simulink model "mpcACCsystem"  (R2023a)
settings: Solver=FixedStepAuto  StartTime=0.0  StopTime=T  RelTol=1e-3
values from neighbouring files (symbols this model uses):
  t_gap = 1.4    [AdaptiveCruiseControlExample.m]
  Ts = 0.1    [AdaptiveCruiseControlExample.m]
  v0_ego = 20    [AdaptiveCruiseControlExample.m]
  v0_lead = 25    [AdaptiveCruiseControlExample.m]
  v_set = 30    [AdaptiveCruiseControlExample.m]
  x0_ego = 10    [AdaptiveCruiseControlExample.m]
  x0_lead = 50    [AdaptiveCruiseControlExample.m]
undefined symbols (not defined in the file or in its folder): MinVelocity
libraries: mpcsigdimcheck_private x10, mpclib x1
settings Model: Creator=The MathWorks, Inc.  LastModifiedBy=15359
settings SolverCC: AlgebraicLoopSolver=TrustRegion
settings DataIOCC: ReturnWorkspaceOutputs=off
settings DebuggingCC: UnconnectedInputMsg=warning  UnconnectedOutputMsg=warning  UnconnectedLineMsg=warning  ArithmeticOperatorsInVariantConditions=warning
settings ModelReferenceCC: EnableRefExpFcnMdlSchedulingChecks=on
settings SFSimCC: SimUseLocalCustomCode=off  CustomCodeUndefinedFunction=UseInterfaceOnly
settings RTWCC: RTWUseLocalCustomCode=off
settings CodeAppCC: StateflowObjectComments=on

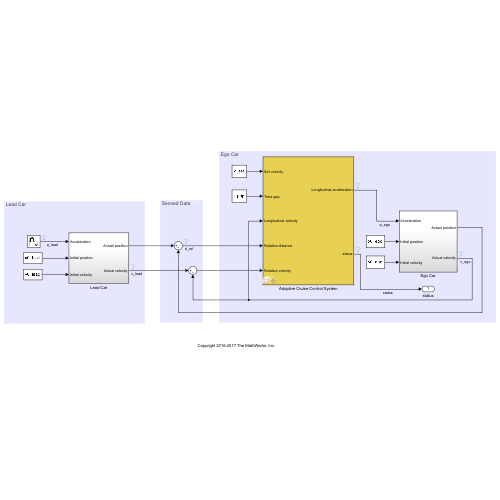
[thumbnail: Simulink's stored preview of the top-level diagram]
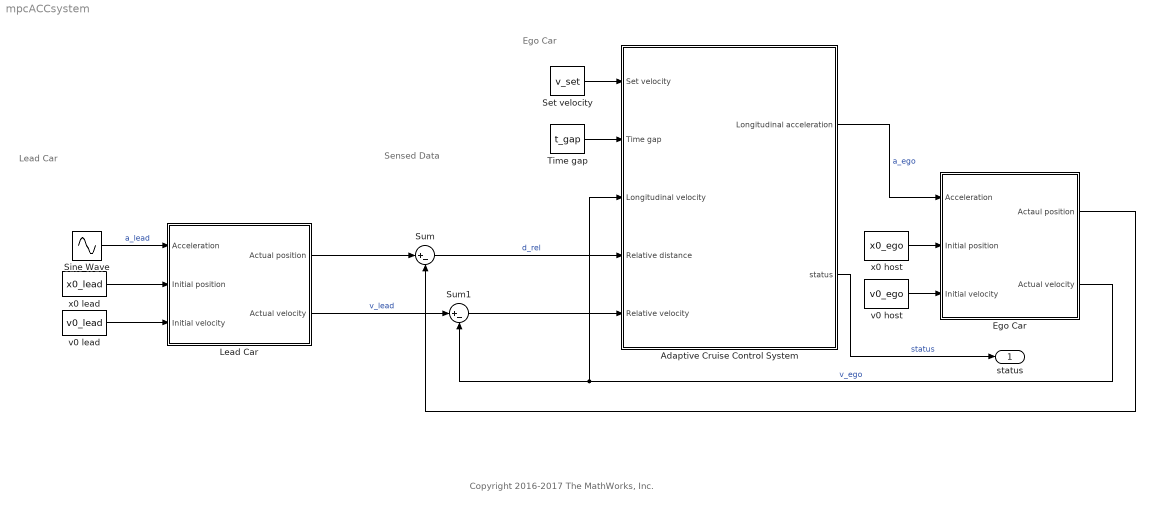
== system mpcACCsystem ==
  note: Sensed Data
  note: Lead Car
  note: Ego Car
  note: Copyright 2016-2017 The MathWorks, Inc.
  Adaptive Cruise Control System : Subsystem  AncestorBlock=mpcadaslib/Adaptive Cruise Control System  mask(Adaptive cruise control (ACC) system){EgoModel=tf(1,[0.5,1,0]), InitialEgoVelocity=20, DefaultSpacing=10, MaxVelocity=50, MinAcceleration=-3, amin_ext=off, MaxAcceleration=2, amax_ext=off, Ts=0.1, PredictionHorizon=30, ControllerBehavior=0.5, suboptimal=off, maxiter=10, datatypeopt=double, optmode=off, trackmode=off}
      mask prompts: EgoModel "MPC:adasblocks:promptACCLinearModel"; InitialEgoVelocity "MPC:adasblocks:promptACCInitialEgoVelocity"; DefaultSpacing "MPC:adasblocks:promptACCDefaultSpacing"; MaxVelocity "MPC:adasblocks:promptACCMaxVelocity"; MinAcceleration "MPC:adasblocks:promptACCMinAcceleration"; amin_ext "MPC:adasblocks:promptACCUseExternalSource"; MaxAcceleration "MPC:adasblocks:promptACCMaxAcceleration"; amax_ext "MPC:adasblocks:promptACCUseExternalSource"; Ts "MPC:adasblocks:promptACCSampleTime"; PredictionHorizon "MPC:adasblocks:promptACCPredictionSteps"; suboptimal "MPC:adasblocks:promptACCUseSubOptimal"; maxiter "MPC:adasblocks:promptACCMaxIter"; datatypeopt "MPC:adasblocks:promptACCDataType"; optmode "MPC:adasblocks:promptACCMPCOptimize"; trackmode "MPC:adasblocks:promptACCSmoothTransition"
      mask help: MPC:adasblocks:accMaskDescription
      mask init:
      | [mpcobj,MinVelocity,DataType] = accblock_MaskInitFcn(gcb,EgoModel,DefaultSpacing,MaxVelocity,...
      |                                                                     MaxAcceleration,MinAcceleration,...
      |                                                                     InitialEgoVelocity,...
      |                                                                     PredictionHorizon,Ts,maxiter,ControllerBehavior);
      settings: LibrarySourceBlock=mpcadaslib/Adaptive Cruise Control System
      mask Help: eval('mpcCSHelp(''mpcBlockACC'')');
      mask Callback amin_ext: adasblocks_utilUseExternal(gcb,'MinAcceleration','amin_ext');
      mask Callback amax_ext: adasblocks_utilUseExternal(gcb,'MaxAcceleration','amax_ext');
      mask Callback suboptimal: adasblocks_callbackUsesuboptimal(gcb);
      mask TypeOptions datatypeopt: double | single
      mask DialogControl DescTextVar Tooltip: MPC:adasblocks:ttipACCMaskDescription
      mask DialogControl Container18 Prompt: MPC:adasblocks:promptACCTabParameters
      mask DialogControl Container30 Prompt: MPC:adasblocks:promptACCEgoVehicle
      mask DialogControl EgoModel Prompt: Linear model from longitudinal acceleration to longitudinal velocity
      mask DialogControl EgoModel Tooltip: MPC:adasblocks:ttipACCLinearModel
      mask DialogControl InitialEgoVelocity Prompt: Initial condition for longitudinal velocity (m/s)
      mask DialogControl InitialEgoVelocity Tooltip: MPC:adasblocks:ttipACCInitialEgoVelocity
      mask DialogControl DefaultSpacing Prompt: Default spacing (m)
      mask DialogControl DefaultSpacing Tooltip: MPC:adasblocks:ttipACCDefaultSpacing
      mask DialogControl MaxVelocity Prompt: Maximum velocity (m/s)
      mask DialogControl MaxVelocity Tooltip: MPC:adasblocks:ttipACCMaxVelocity
      mask DialogControl Container22 Prompt: MPC:adasblocks:promptACCConstraints
      mask DialogControl MinAcceleration Prompt: Minimum longitudinal acceleration (m/s^2)
      mask DialogControl MinAcceleration Tooltip: MPC:adasblocks:ttipACCMaxDeceleration
      mask DialogControl amin_ext Prompt: Use external source
      mask DialogControl MaxAcceleration Prompt: Maximum longitudinal acceleration (m/s^2)
      mask DialogControl MaxAcceleration Tooltip: MPC:adasblocks:ttipACCMaxAcceleration
      mask DialogControl amax_ext Prompt: Use external source
      mask DialogControl Container9 Prompt: MPC:adasblocks:promptACCMPCSettings
      mask DialogControl Ts Prompt: Sample time (s)
      mask DialogControl Ts Tooltip: MPC:adasblocks:ttipACCSampleTime
      mask DialogControl PredictionHorizon Prompt: Prediction horizon (steps)
      mask DialogControl PredictionHorizon Tooltip: MPC:adasblocks:ttipACCPredictionSteps
      mask DialogControl Container14 Prompt: MPC:adasblocks:promptACCWeight
      mask DialogControl ControllerBehavior Tooltip: MPC:adasblocks:ttipACCWeight
      mask DialogControl SliderText Prompt: More robust            More aggressive
      mask DialogControl Container21 Prompt: MPC:adasblocks:promptACCOptionsText
      mask DialogControl Container19 Prompt: MPC:adasblocks:promptACCOptimization
      mask DialogControl suboptimal Prompt: Use suboptimal solution
      mask DialogControl suboptimal Tooltip: MPC:adasblocks:ttipACCUseSubOptimal
      mask DialogControl maxiter Prompt: Maximum iteration number
      mask DialogControl maxiter Tooltip: MPC:adasblocks:ttipACCMaxIter
      mask DialogControl datatypeopt Prompt: Data Type
      mask DialogControl datatypeopt Tooltip: MPC:adasblocks:ttipACCDataType
      mask DialogControl Container23 Prompt: MPC:adasblocks:promptACCBlockOptions
      mask DialogControl optmode Prompt: Use external signal to enable or disable optimization
      mask DialogControl optmode Tooltip: MPC:adasblocks:ttipACCMPCOptimize
      mask DialogControl trackmode Prompt: Use external control signal for bumpless transfer between ACC and other controllers
      mask DialogControl trackmode Tooltip: MPC:adasblocks:ttipACCSmoothTransition
      mask DialogControl Container25 Prompt: MPC:adasblocks:promptACCCustomizeText
      mask DialogControl Control7 Prompt: MPC:adasblocks:promptACCCreateSystemTextMore
      mask DialogControl Control3 Prompt: MPC:adasblocks:promptACCCreateSysBtn
      mask DialogControl Control3 Tooltip: MPC:adasblocks:ttipACCCreateSysBtn
      mask DialogControl Control3 Callback: accblock_callbackCreateSubsystemButton(gcb);
  Ego Car : Subsystem
  Lead Car : Subsystem
  Set velocity : Constant  Value=v_set  SampleTime=Ts
  Sine Wave : Sin  Amplitude=0.6  Frequency=0.2  SampleTime=Ts
  Sum : Sum  Inputs=|+-
  Sum1 : Sum  Inputs=|+-
  Time gap : Constant  Value=t_gap  SampleTime=Ts
  v0 host : Constant  Value=v0_ego  SampleTime=Ts
  v0 lead : Constant  Value=v0_lead  SampleTime=Ts
  x0 host : Constant  Value=x0_ego  SampleTime=Ts
  x0 lead : Constant  Value=x0_lead  SampleTime=Ts
  status : Outport
  wires:
  x0 lead/1 -> Lead Car/2(Initial position)
  v0 lead/1 -> Lead Car/3(Initial velocity)
  x0 host/1 -> Ego Car/2(Initial position)
  Ego Car/1(Actaul position) -> Sum/2
  Ego Car/2(Actual velocity) -> Adaptive Cruise Control System/3(Longitudinal velocity), Sum1/2  "v_ego"
  v0 host/1 -> Ego Car/3(Initial velocity)
  Set velocity/1 -> Adaptive Cruise Control System/1(Set velocity)
  Adaptive Cruise Control System/1(Longitudinal acceleration) -> Ego Car/1(Acceleration)  "a_ego"
  Lead Car/1(Actual position) -> Sum/1
  Sum1/1 -> Adaptive Cruise Control System/5(Relative velocity)
  Time gap/1 -> Adaptive Cruise Control System/2(Time gap)
  Sine Wave/1 -> Lead Car/1(Acceleration)  "a_lead"
  Lead Car/2(Actual velocity) -> Sum1/1  "v_lead"
  Sum/1 -> Adaptive Cruise Control System/4(Relative distance)  "d_rel"
  Adaptive Cruise Control System/2(status) -> status/1  "status"

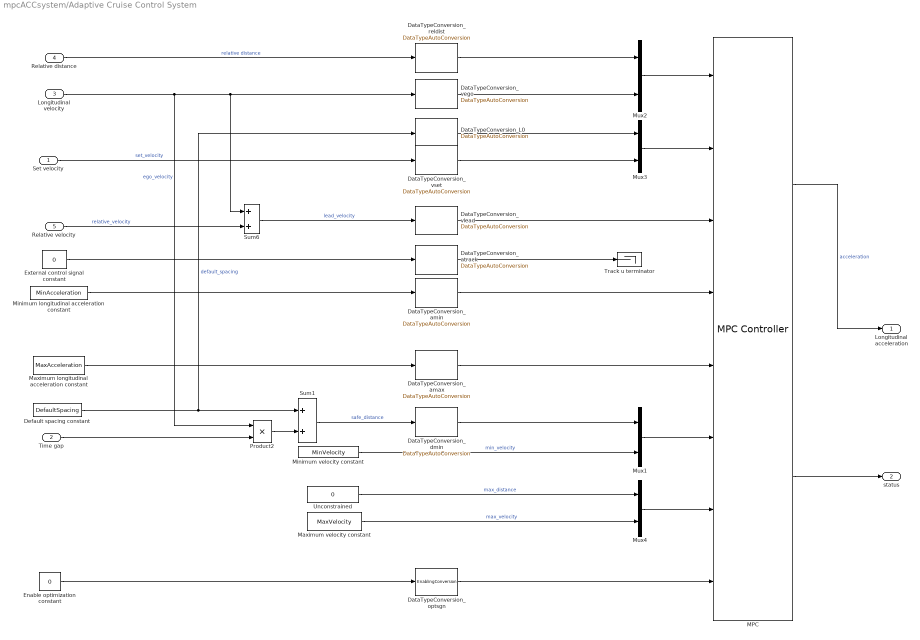
== system mpcACCsystem/Adaptive Cruise Control System ==
  Set velocity : Inport
  Time gap : Inport  Port=2
  Longitudinal velocity : Inport  Port=3
  Relative distance : Inport  Port=4
  Relative velocity : Inport  Port=5
  DataTypeConversion_L0 : mpcsigdimcheck_private/DataTypeAutoConversion  datatypestr=DataType
  DataTypeConversion_amax : mpcsigdimcheck_private/DataTypeAutoConversion  datatypestr=DataType
  DataTypeConversion_amin : mpcsigdimcheck_private/DataTypeAutoConversion  datatypestr=DataType
  DataTypeConversion_atrack : mpcsigdimcheck_private/DataTypeAutoConversion  datatypestr=DataType
  DataTypeConversion_dmin : mpcsigdimcheck_private/DataTypeAutoConversion  datatypestr=DataType
  DataTypeConversion_optsgn : mpcsigdimcheck_private/EnablingConversion  SystemSampleTime=-1  VariantActivationTime=update diagram  Latency=0  AutoFrameSizeCalculation=off
  DataTypeConversion_reldist : mpcsigdimcheck_private/DataTypeAutoConversion  datatypestr=DataType
  DataTypeConversion_vego : mpcsigdimcheck_private/DataTypeAutoConversion  datatypestr=DataType
  DataTypeConversion_vlead : mpcsigdimcheck_private/DataTypeAutoConversion  datatypestr=DataType
  DataTypeConversion_vset : mpcsigdimcheck_private/DataTypeAutoConversion  datatypestr=DataType
  Default spacing constant : Constant  Value=DefaultSpacing
  Enable optimization constant : Constant  Value=0
  External control signal constant : Constant  Value=0  OutDataTypeStr=double
  MPC : mpclib/MPC Controller  SCDEnableBlockLinearizationSpecification=on  mpcobj=mpcobj  is_multiple=0  enable_value=0  return_u0=off  updateMPCinCallerWorkspace=off  md_inport=on  mv_inport=off  uref_inport=off  return_cost=off  return_mvseq=off  return_qpstatus=on  return_xseq=off  return_state=off  return_ovseq=off  state_inport=off  umin_inport=on  umax_inport=on  ymin_inport=on  ymax_inport=on  cc_inport=off  ywt_inport=off  uwt_inport=off  duwt_inport=off  rhoeps_inport=off  pm_inport=off  MaximumP=10  HorizonChoice=FixedHorizon  n_ts=0.1  n_p=30  n_mv=1  n_md=1  n_ud=0  n_mo=2  n_uo=0  BlockDataType=double  SampleTimeInherited=off  switch_inport=on
  Maximum longitudinal acceleration constant : Constant  Value=MaxAcceleration
  Maximum velocity constant : Constant  Value=MaxVelocity  OutDataTypeStr=DataType
  Minimum longitudinal acceleration constant : Constant  Value=MinAcceleration
  Minimum velocity constant : Constant  Value=MinVelocity  OutDataTypeStr=DataType
  Mux{1..4} (4 alike) : Mux  Inputs=[1 1]
  Product2 : Product
  Sum1 : Sum
  Sum6 : Sum
  Track u terminator : Terminator
  Unconstrained : Constant  Value=0  OutDataTypeStr=DataType
  Longitudinal acceleration : Outport  PortDimensions=1  VectorParamsAs1DForOutWhenUnconnected=off
  status : Outport  Port=2  PortDimensions=1  VectorParamsAs1DForOutWhenUnconnected=off
  wires:
  DataTypeConversion_atrack/1 -> Track u terminator/1
  External control signal constant/1 -> DataTypeConversion_atrack/1
  DataTypeConversion_optsgn/1 -> MPC/8
  Enable optimization constant/1 -> DataTypeConversion_optsgn/1
  Unconstrained/1 -> Mux4/1  "max_distance"
  Maximum velocity constant/1 -> Mux4/2  "max_velocity"
  Mux4/1 -> MPC/7
  Maximum longitudinal acceleration constant/1 -> DataTypeConversion_amax/1
  Minimum longitudinal acceleration constant/1 -> DataTypeConversion_amin/1
  Set velocity/1 -> DataTypeConversion_vset/1  "set_velocity"
  Time gap/1 -> Product2/2
  DataTypeConversion_vego/1 -> Mux2/2
  DataTypeConversion_reldist/1 -> Mux2/1
  DataTypeConversion_vset/1 -> Mux3/2
  DataTypeConversion_L0/1 -> Mux3/1
  DataTypeConversion_vlead/1 -> MPC/3
  DataTypeConversion_dmin/1 -> Mux1/1
  DataTypeConversion_amin/1 -> MPC/4
  DataTypeConversion_amax/1 -> MPC/5
  Mux1/1 -> MPC/6
  Sum1/1 -> DataTypeConversion_dmin/1  "safe_distance"
  Minimum velocity constant/1 -> Mux1/2  "min_velocity"
  Product2/1 -> Sum1/2
  MPC/1 -> Longitudinal acceleration/1  "acceleration"
  Relative velocity/1 -> Sum6/2  "relative_velocity"
  Relative distance/1 -> DataTypeConversion_reldist/1  "relative distance"
  Longitudinal velocity/1 -> Sum6/1, DataTypeConversion_vego/1, Product2/1  "ego_velocity"
  Mux3/1 -> MPC/2
  Mux2/1 -> MPC/1
  Default spacing constant/1 -> Sum1/1, DataTypeConversion_L0/1  "default_spacing"
  Sum6/1 -> DataTypeConversion_vlead/1  "lead_velocity"
  MPC/2 -> status/1

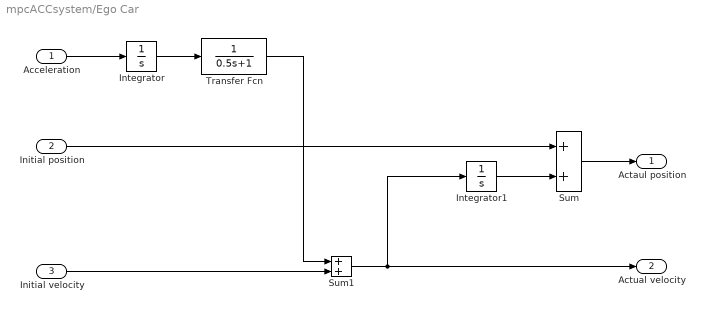
== system mpcACCsystem/Ego Car ==
  Acceleration : Inport
  Initial position : Inport  Port=2
  Initial velocity : Inport  Port=3
  Integrator : Integrator
  Integrator1 : Integrator
  Sum : Sum
  Sum1 : Sum
  Transfer Fcn : TransferFcn  Denominator=[0.5 1]
  Actaul position : Outport  VectorParamsAs1DForOutWhenUnconnected=off
  Actual velocity : Outport  Port=2  VectorParamsAs1DForOutWhenUnconnected=off
  wires:
  Sum1/1 -> Integrator1/1, Actual velocity/1
  Initial velocity/1 -> Sum1/2
  Sum/1 -> Actaul position/1
  Transfer Fcn/1 -> Sum1/1
  Integrator/1 -> Transfer Fcn/1
  Acceleration/1 -> Integrator/1
  Initial position/1 -> Sum/1
  Integrator1/1 -> Sum/2

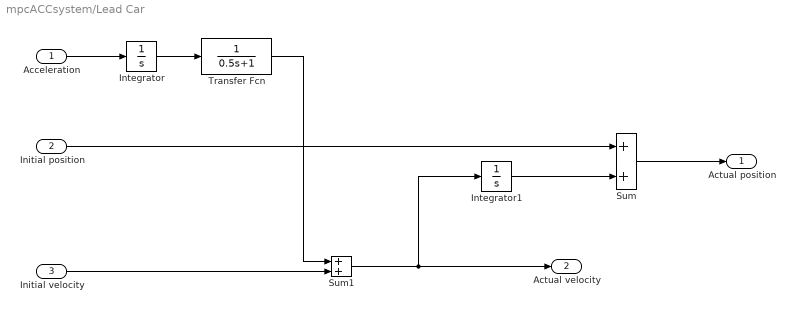
== system mpcACCsystem/Lead Car ==
  Acceleration : Inport
  Initial position : Inport  Port=2
  Initial velocity : Inport  Port=3
  Integrator : Integrator
  Integrator1 : Integrator
  Sum : Sum
  Sum1 : Sum
  Transfer Fcn : TransferFcn  Denominator=[0.5 1]
  Actual position : Outport  VectorParamsAs1DForOutWhenUnconnected=off
  Actual velocity : Outport  Port=2  VectorParamsAs1DForOutWhenUnconnected=off
  wires:
  Transfer Fcn/1 -> Sum1/1
  Initial velocity/1 -> Sum1/2
  Sum/1 -> Actual position/1
  Integrator/1 -> Transfer Fcn/1
  Sum1/1 -> Integrator1/1, Actual velocity/1
  Acceleration/1 -> Integrator/1
  Initial position/1 -> Sum/1
  Integrator1/1 -> Sum/2
